simulink model "Microgrid_W"  (R2020a)
settings: Solver=ode15s  StartTime=0  StopTime=1440*1  MaxStep=1  RelTol=1e-3
libraries: simulink x4214, powerlib x685, simulink_extras x28, Microgrid_Library x18, powerlib_meascontrol x12
(part 48 of 48)

== system Microgrid_W/House 5 W2/Refrigerator/Subsystem/Thermostat ==
  In1 : Inport
  Compare To Constant : simulink/Logic and Bit Operations/Compare To Constant  relop=>=  const=T_High  OutDataTypeStr=boolean
  Compare To Constant1 : simulink/Logic and Bit Operations/Compare To Constant  relop=<=  const=T_Low  OutDataTypeStr=boolean
  Constant : Constant  Value=0
  Constant1 : Constant
  S-R Flip-Flop : simulink_extras/Flip Flops/S-R Flip-Flop  initial_condition=0
  Switch : Switch  Criteria=u2 > Threshold  Threshold=0.5
  Out1 : Outport  VectorParamsAs1DForOutWhenUnconnected=off
  wires:
  Constant1/1 -> Switch/3
  Constant/1 -> Switch/1
  Switch/1 -> Out1/1
  S-R Flip-Flop/1 -> Switch/2
  Compare To Constant1/1 -> S-R Flip-Flop/1
  Compare To Constant/1 -> S-R Flip-Flop/2
  In1/1 -> Compare To Constant/1, Compare To Constant1/1

== system Microgrid_W/House 5 W3/Refrigerator/Subsystem/Thermostat ==
  In1 : Inport
  Compare To Constant : simulink/Logic and Bit Operations/Compare To Constant  relop=>=  const=T_High  OutDataTypeStr=boolean
  Compare To Constant1 : simulink/Logic and Bit Operations/Compare To Constant  relop=<=  const=T_Low  OutDataTypeStr=boolean
  Constant : Constant  Value=0
  Constant1 : Constant
  S-R Flip-Flop : simulink_extras/Flip Flops/S-R Flip-Flop  initial_condition=0
  Switch : Switch  Criteria=u2 > Threshold  Threshold=0.5
  Out1 : Outport  VectorParamsAs1DForOutWhenUnconnected=off
  wires:
  In1/1 -> Compare To Constant1/1, Compare To Constant/1
  Compare To Constant/1 -> S-R Flip-Flop/2
  Compare To Constant1/1 -> S-R Flip-Flop/1
  S-R Flip-Flop/1 -> Switch/2
  Switch/1 -> Out1/1
  Constant/1 -> Switch/1
  Constant1/1 -> Switch/3

== matlab function Microgrid_W/House 2 W1/House 2 Controller1 ==
  data: T_HIGH input; HW_W input; D output; solar input; T input
function D = fcn(T_HIGH, HW_W, solar, T)
    

    unused_solar = solar;
    if isnan(unused_solar)
        unused_solar = 0;
    end

    if (unused_solar >= HW_W)
        D = 1.0;
    else 
        D = unused_solar / HW_W;
    end

== matlab function Microgrid_W/House 3 W1/House 2 Controller1 ==
  data: HW_W input; D output; solar input
function D = fcn(HW_W, solar)
    unused_solar = solar;
    if isnan(unused_solar)
        unused_solar = 0;
    end

    if (unused_solar >= HW_W)
        D = 1.0;
    else 
        D = unused_solar / HW_W;
    end

== matlab function Microgrid_W/House 4 W1/House 2 Controller1 ==
  data: HW_W input; D output; solar input
function D = fcn(HW_W, solar)
    unused_solar = solar;
    if isnan(unused_solar)
        unused_solar = 0;
    end

    if (unused_solar >= HW_W)
        D = 1.0;
    else 
        D = unused_solar / HW_W;
    end

== matlab function Microgrid_W/House 5 W1/House 2 Controller1 ==
  data: HW_W input; D output; solar input
function D = fcn(HW_W, solar)
    unused_solar = solar;
    if isnan(unused_solar)
        unused_solar = 0;
    end

    if (unused_solar >= HW_W)
        D = 1.0;
    else 
        D = unused_solar / HW_W;
    end

== matlab function Microgrid_W/House 2 W3/House 2 Controller1 ==
  data: thermo input; sw output; solar input
function sw = fcn(thermo, solar)
    if (solar > 0) && (thermo > 0)
        sw =1;
    else 
        sw = 0;
    end

== matlab function Microgrid_W/House 3 W3/House 3 Controller1 ==
  data: thermo input; sw output; solar input
function sw = fcn(thermo, solar)
    if (solar > 0) && (thermo > 0)
        sw =1;
    else 
        sw = 0;
    end

== matlab function Microgrid_W/House 4 W3/House 4 Controller1 ==
  data: thermo input; sw output; solar input
function sw = fcn(thermo, solar)
    if (solar > 0) && (thermo > 0)
        sw =1;
    else 
        sw = 0;
    end

== matlab function Microgrid_W/House 5 W3/House 5 Controller1 ==
  data: thermo input; sw output; solar input
function sw = fcn(thermo, solar)
    if (solar > 0) && (thermo > 0)
        sw = 1;
    else 
        sw = 0;
    end
